simulink model "Latest_HIWI_model"  (R2023b)
settings: Solver=VariableStepAuto  StartTime=0*24*3600  StopTime=24*3600*3  MaxStep=60  RelTol=1e-4  EnableMultiTasking=on
values from neighbouring files (symbols this model uses):
  C_Battery_kWh = 80    [workspaceHIWI.mat]
  discharge_car = [0 3600 7200 10800 14400 18000 21600 25200 28800 32400 36000 39600 ... (146 elements, 73x2)]    [workspaceHIWI.mat]
  Max_charge_potential = 5000    [workspaceHIWI.mat]
  P_Inv_W_max = 12000    [workspaceHIWI.mat]
  PV_W = 10000    [workspaceHIWI.mat]
  ReqSOCandtime1 = [0 3600 7200 10800 14400 18000 21600 25200 28800 32400 36000 39600 ... (219 elements, 73x3)]    [workspaceHIWI.mat]
  SOC_max = 1    [workspaceHIWI.mat]
  SOC_min = 0.1    [workspaceHIWI.mat]
undefined symbols (not defined in the file or in its folder): Davies, Hay, path_carnot, phase
libraries: carnot x11
settings Model: Creator=drhf  LastModifiedBy=Rohan
settings SolverCC: AlgebraicLoopSolver=TrustRegion  EnableFixedStepZeroCrossing=on
settings DataIOCC: LimitDataPoints=on  SaveFormat=Array  ReturnWorkspaceOutputs=off
settings OptimizationCC: ExpressionDepthLimit=2147483647  LifeSpan=inf
settings DebuggingCC: AlgebraicLoopMsg=none  UnderspecifiedInitializationDetection=Classic  MergeDetectMultiDrivingBlocksExec=none  SolverPrmCheckMsg=warning  FcnCallInpInsideContextMsg=warning  UnconnectedInputMsg=warning  UnconnectedOutputMsg=warning  UnconnectedLineMsg=warning  StateNameClashWarn=warning  SFUnexpectedBacktrackingDiag=warning  SFNoUnconditionalDefaultTransitionDiag=warning  SFExecutionAtInitializationDiag=none  ArithmeticOperatorsInVariantConditions=warning
settings HardwareCC: ProdBitPerPointer=32  ProdBitPerSizeT=32  ProdBitPerPtrDiffT=32  ProdLargestAtomicFloat=None  ProdIntDivRoundTo=Undefined  ProdEndianess=Unspecified  ProdWordSize=32  ProdHWDeviceType=32-bit Generic
settings ModelReferenceCC: EnableRefExpFcnMdlSchedulingChecks=on  PropagateSignalLabelsOutOfModel=off
settings SFSimCC: SimUseLocalCustomCode=off  CustomCodeUndefinedFunction=UseInterfaceOnly
settings RTWCC: RTWUseLocalCustomCode=off
settings CodeAppCC: StateflowObjectComments=on
settings GRTTargetCC: TargetLangStandard=C89/C90 (ANSI)  CombineOutputUpdateFcns=off  GRTInterface=on
settings ConfigComp: CovMetricSettings=dw  CovSaveCumulativeToWorkspaceVar=on  CovSaveSingleToWorkspaceVar=on  CovExternalEMLEnable=off

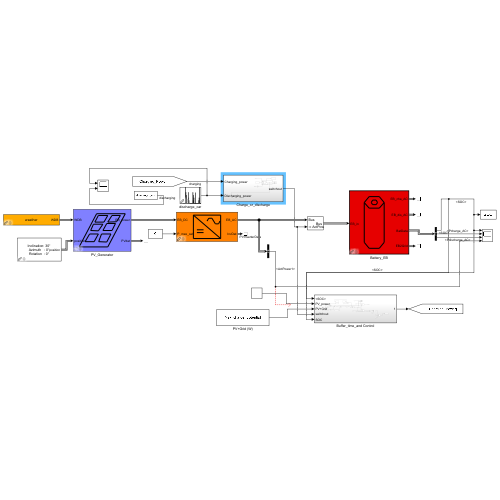
[thumbnail: Simulink's stored preview of the top-level diagram]
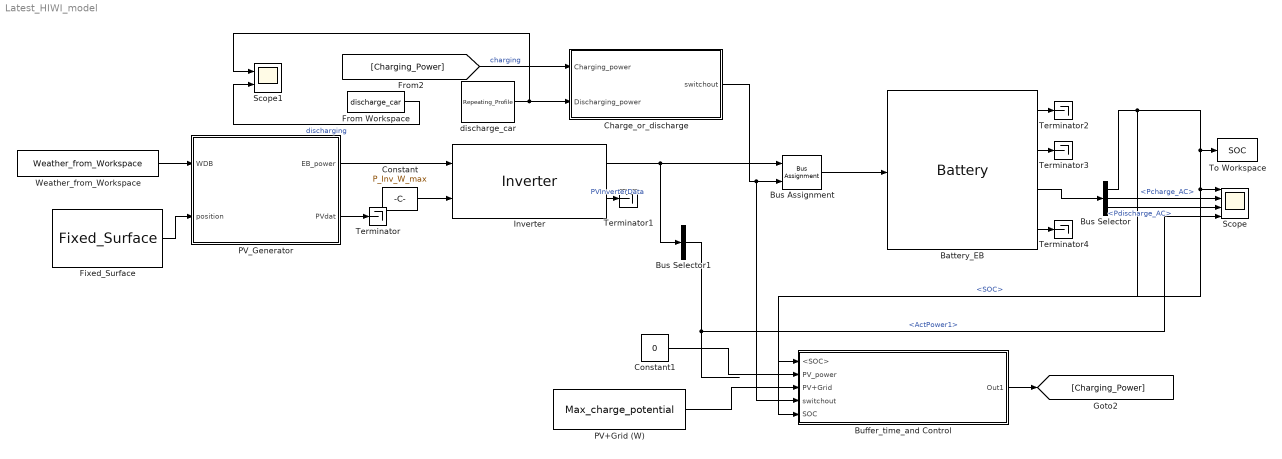
== system Latest_HIWI_model ==
  Battery_EB : carnot/Storage/Electric/Battery  cap_kWh=C_Battery_kWh  eta_ch=n_Charge  eta_dis=n_Discharge  cap0=(SOC_max+SOC_min)/2  SOC_max=SOC_max  SOC_min=SOC_min  Pmax=P_Charge_W  Pmin=P_Discharge_W  P_standby=0
  Buffer_time_and Control : Subsystem
  Bus Assignment : BusAssignment  AssignedSignals=ActPower1
  Bus Selector : BusSelector  OutputSignals=SOC,Pcharge_AC,Pdischarge_AC
  Bus Selector1 : BusSelector  OutputSignals=ActPower1
  Charge_or_discharge : Subsystem
  Constant : Constant  Value=P_Inv_W_max
  Constant1 : Constant  Value=0
  Fixed_Surface : carnot/Weather/Fixed_Surface  colangle=30  colazi=0  colrot=0
  From Workspace : FromWorkspace  VariableName=discharge_car
  Inverter : carnot/Source/Electric_Generator/Inverter  PathName=fullfile(path_carnot('libsl'), 'Source','Electric_Generator','Inverter','parameter_set')  FileName='<user defined>'  userPath=off  userParam=on  Pacnom=P_Inv_W  nphase=1-phase  U=230  f=50  PstepsEta=[0 0.1 0.2 0.25 0.3 0.5 0.75 1]  Eta=[0 0.948 0.966 0.969 0.97 0.972 0.97 0.967]  P_standby=2
  PV+Grid (W) : Constant  Value=Max_charge_potential
  PV_Generator : Subsystem  AncestorBlock=carnot/Source/Electric_Generator/PV_Generator  mask(PV_Module_simple){Wp=PV_W, delta_Wp_K=0.0047, fgen=0.91 % 0.06 power missmatch, 0.01 diodes, 0.02 data sheet tolerance}
      mask prompts: Wp "Peak power of the generator [W]"; delta_Wp_K "Temperature coefficient Pmax 1/K"; fgen "efficiency generator field (lossses in diodes, power missmatch, dirt)"
      mask help:
      | This block simultes a PV module or generatater and calculates the DC power based on the parameters:
      | - Wp of one module or generator at STC [W]
      | - temperature coefficient of Pmax [1/K]
      | - dirt and degradation effects
      | The output DC power of the PV generator is ActPower1 in EB (power only)
      mask Help: web(fullfile(path_carnot('help'),'PV_Generator.html'),'-helpbrowser')
      mask Display: plot(0,0,100,100,[10,40,90,60,10],[10,90,90,10,10],[37,53,60,43,37],[70,70,86,86,70],[60,75,82,67,60],[70,71,86,86,70],[35,30,43,51,35],[65,50,49,65,65],[51,67,73,58,51],[50,50,66,66,50],[28,20,36,43,28],[41,23,23,41,41],[49,44,58,65,49],[41,23,22,41,41])
  Scope : Scope  NumInputPorts=4
  Scope1 : Scope  NumInputPorts=2
  Terminator{,1..4} (5 alike) : Terminator
  To Workspace : ToWorkspace  VariableName=SOC  SampleTime=-1
  Weather_from_Workspace : carnot/Weather/Weather_from_Workspace  file=weather
  discharge_car : carnot/Load/General/Repeating_Profile  period=discharge_car(end,1)  rep_seq_t=discharge_car(:,1)'  rep_seq_d=[1 ]*3600  rep_seq_y=discharge_car(:,2)'
  wires:
  PV_Generator/1(EB_power) -> Inverter/1
  Fixed_Surface/1 -> PV_Generator/2(position)
  Weather_from_Workspace/1 -> PV_Generator/1(WDB)
  PV_Generator/2(PVdat) -> Terminator/1
  Constant/1 -> Inverter/2
  Inverter/2 -> Terminator1/1  "PVInverterData"
  Bus Assignment/1 -> Battery_EB/1
  Inverter/1 -> Bus Selector1/1, Bus Assignment/1
  Battery_EB/3 -> Bus Selector/1
  Bus Selector/1 -> Buffer_time_and Control/5(SOC), Scope/1, To Workspace/1, Buffer_time_and Control/1(<SOC>)  "<SOC>"
  Bus Selector1/1 -> Scope/4  "<ActPower1>"
  Bus Selector/2 -> Scope/2  "<Pcharge_AC>"
  Bus Selector/3 -> Scope/3  "<Pdischarge_AC>"
  Battery_EB/1 -> Terminator2/1
  Battery_EB/2 -> Terminator3/1
  Battery_EB/4 -> Terminator4/1
  Buffer_time_and Control/1(Out1) -> [Charging_Power]
  Charge_or_discharge/1(switchout) -> Buffer_time_and Control/4(switchout), Bus Assignment/2
  [Charging_Power] -> Charge_or_discharge/1(Charging_power)  "charging"
  From Workspace/1 -> Scope1/2  "discharging"
  PV+Grid (W)/1 -> Buffer_time_and Control/3(PV+Grid)
  discharge_car/1 -> Scope1/1, Charge_or_discharge/2(Discharging_power)
  Constant1/1 -> Buffer_time_and Control/2(PV_power)

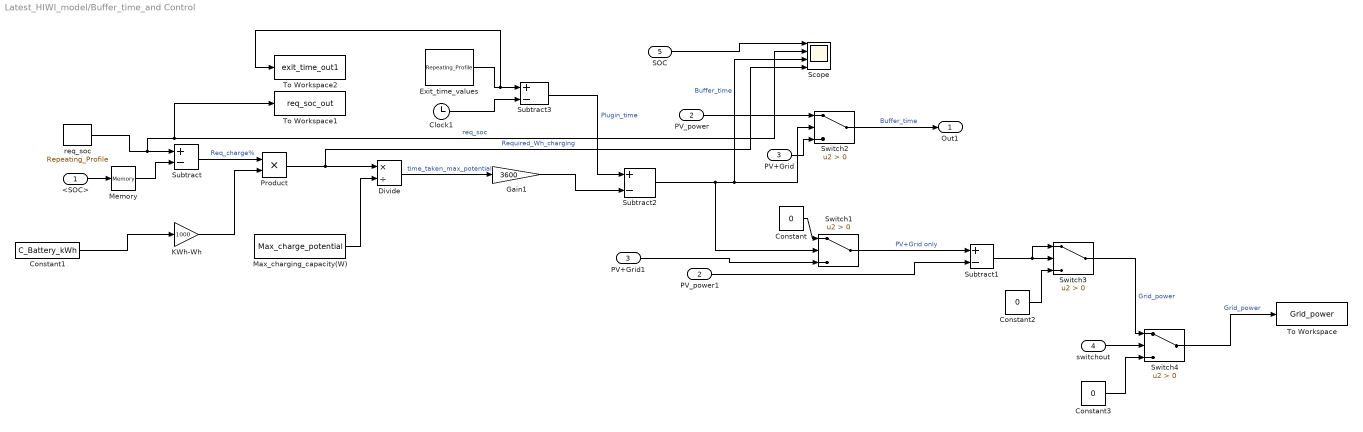
== system Latest_HIWI_model/Buffer_time_and Control ==
  <SOC> : Inport
  PV_power : Inport  Port=2
  PV+Grid : Inport  Port=3
  switchout : Inport  Port=4
  SOC : Inport  Port=5
  Clock1 : Clock
  Constant : Constant  Value=0
  Constant1 : Constant  Value=C_Battery_kWh
  Constant2 : Constant  Value=0
  Constant3 : Constant  Value=0
  Divide : Product  Inputs=*/
  Exit_time_values : carnot/Load/General/Repeating_Profile  period=ReqSOCandtime1(end,1)  rep_seq_t=ReqSOCandtime1(:,1)'  rep_seq_d=[1 ]*3600  rep_seq_y=ReqSOCandtime1(:,3)'
  Gain1 : Gain  Gain=3600
  KWh-Wh : Gain  Gain=1000
  Max_charging_capacity(W) : Constant  Value=Max_charge_potential
  Memory : Memory  InitialCondition=0.55
  PV+Grid1 : InportShadow  Port=3
  PV_power1 : InportShadow  Port=2
  Product : Product
  Scope : Scope  NumInputPorts=4
  Subtract{,1..3} (4 alike) : Sum  Inputs=+-
  Switch{1..4} (4 alike) : Switch  Criteria=u2 > Threshold  SaturateOnIntegerOverflow=off  InputSameDT=off
  To Workspace : ToWorkspace  VariableName=Grid_power  SampleTime=-1
  To Workspace1 : ToWorkspace  VariableName=req_soc_out  SaveFormat=Timeseries  SampleTime=-1
  To Workspace2 : ToWorkspace  VariableName=exit_time_out1  SaveFormat=Timeseries  SampleTime=-1
  req_soc : carnot/Load/General/Repeating_Profile  period=ReqSOCandtime1(end,1)  rep_seq_t=ReqSOCandtime1(:,1)'  rep_seq_d=[1 ]*3600  rep_seq_y=ReqSOCandtime1(:,2)'
  Out1 : Outport
  wires:
  Subtract3/1 -> Subtract2/1  "Plugin_time"
  KWh-Wh/1 -> Product/2
  Max_charging_capacity(W)/1 -> Divide/2
  Subtract2/1 -> Switch1/2, Scope/3, Switch2/2  "Buffer_time"
  Product/1 -> Scope/4, Divide/1  "Required_Wh_charging"
  Subtract/1 -> Product/1  "Req_charge%"
  req_soc/1 -> To Workspace1/1, Scope/2, Subtract/1  "req_soc"
  Exit_time_values/1 -> To Workspace2/1, Subtract3/1
  Gain1/1 -> Subtract2/2
  Divide/1 -> Gain1/1  "time_taken_max_potential"
  Clock1/1 -> Subtract3/2
  Constant1/1 -> KWh-Wh/1
  Switch2/1 -> Out1/1  "Buffer_time"
  <SOC>/1 -> Memory/1
  PV_power/1 -> Switch2/1
  PV+Grid/1 -> Switch2/3
  PV_power1/1 -> Subtract1/2
  PV+Grid1/1 -> Switch1/3
  Subtract1/1 -> Switch3/1, Switch3/2
  Constant2/1 -> Switch3/3
  Switch3/1 -> Switch4/1  "Grid_power"
  Switch1/1 -> Subtract1/1  "PV+Grid only"
  Constant/1 -> Switch1/1
  switchout/1 -> Switch4/2
  Constant3/1 -> Switch4/3
  Switch4/1 -> To Workspace/1  "Grid_power"
  SOC/1 -> Scope/1
  Memory/1 -> Subtract/2

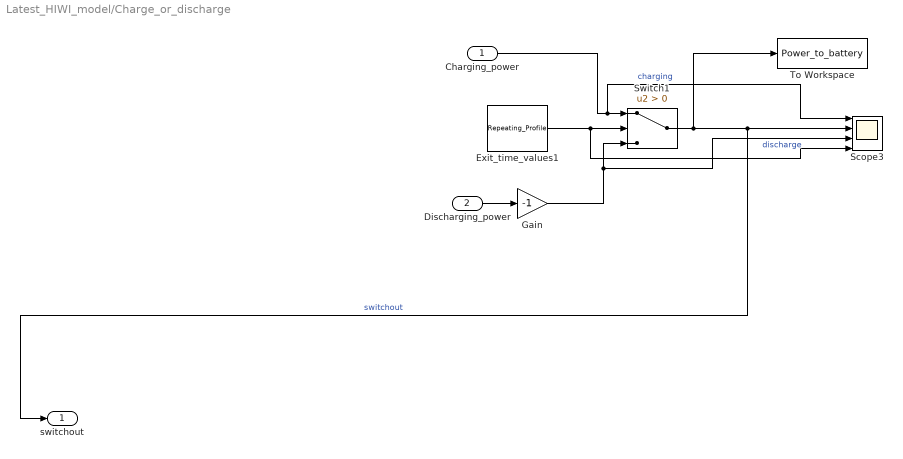
== system Latest_HIWI_model/Charge_or_discharge ==
  Charging_power : Inport
  Discharging_power : Inport  Port=2
  Exit_time_values1 : carnot/Load/General/Repeating_Profile  period=ReqSOCandtime1(end,1)  rep_seq_t=ReqSOCandtime1(:,1)'  rep_seq_d=[1 ]*3600  rep_seq_y=ReqSOCandtime1(:,3)'
  Gain : Gain  Gain=-1
  Scope3 : Scope  NumInputPorts=4
  Switch1 : Switch  Criteria=u2 > Threshold  SaturateOnIntegerOverflow=off  InputSameDT=off  OutDataTypeStr=Inherit: Same as first input
  To Workspace : ToWorkspace  VariableName=Power_to_battery  SaveFormat=Timeseries  SampleTime=-1
  switchout : Outport
  wires:
  Switch1/1 -> To Workspace/1, switchout/1, Scope3/2  "switchout"
  Charging_power/1 -> Scope3/1, Switch1/1  "charging"
  Exit_time_values1/1 -> Scope3/4, Switch1/2
  Gain/1 -> Scope3/3, Switch1/3  "discharge"
  Discharging_power/1 -> Gain/1

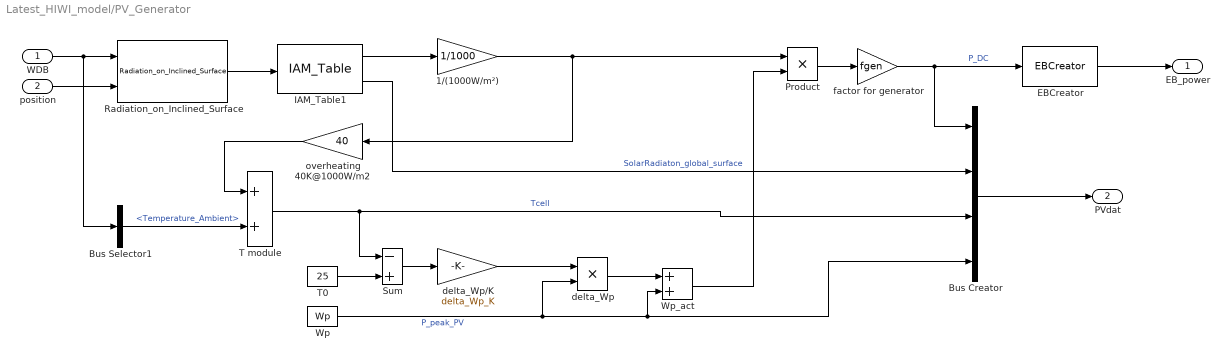
== system Latest_HIWI_model/PV_Generator ==
  WDB : Inport
  position : Inport  Port=2
  1/(1000W/m²) : Gain  Gain=1/1000
  Bus Creator : BusCreator  Inputs=4
  Bus Selector1 : BusSelector  OutputSignals=Temperature_Ambient
  EBCreator : carnot/Basic/Electric/EBCreator  Inport_ID=off  Inport_f=off  Inport_v1=off  Inport_p1=on  Inport_pf1=off  Inport_v2=off  Inport_p2=off  Inport_pf2=off  Inport_v3=off  Inport_p3=off  Inport_pf3=off  ID=1  f=0  v1=0  p1=1e5  pf1=1  v2=0  p2=0  pf2=0  v3=0  p3=0  pf3=0  Annotation_ID=off  Annotation_f=off  Annotation_v1=off  Annotation_p1=off  Annotation_pf1=off  Annotation_v2=off  Annotation_p2=off  Annotation_pf2=off  Annotation_v3=off  Annotation_p3=off  Annotation_pf3=off
  IAM_Table1 : carnot/Source/Solar_Thermal/IncidenceAngleModifier/IAM_Table  fta=1  angle=[0:5:90]  Kb="[1.0000    1.0000    0.9999    0.9996    0.9991    0.9982    0.9965  0.9935    0.9886    0.9807    0.9678    0.9473    0.9148    0.8638   0.7846    0.6644    0.4907    0.2599    0.0000]"  Kd=0.915
  Product : Product  RndMeth=Zero
  Radiation_on_Inclined_Surface : carnot/Weather/Radiation_on_Inclined_Surface  sky=Hay-Davies  reflect=0.2
  Sum : Sum  Inputs=-+
  T module : Sum  Inputs=2
  T0 : Constant  Value=25
  Wp : Constant  Value=Wp
  Wp_act : Sum
  delta_Wp : Product  RndMeth=Zero
  delta_Wp/K : Gain  Gain=delta_Wp_K
  factor for generator : Gain  Gain=fgen
  overheating 40K@1000W/m2 : Gain  Gain=40
  EB_power : Outport  VectorParamsAs1DForOutWhenUnconnected=off
  PVdat : Outport  Port=2  VectorParamsAs1DForOutWhenUnconnected=off
  wires:
  IAM_Table1/2 -> Bus Creator/2  "SolarRadiaton_global_surface"
  position/1 -> Radiation_on_Inclined_Surface/2
  Radiation_on_Inclined_Surface/1 -> IAM_Table1/1
  WDB/1 -> Radiation_on_Inclined_Surface/1, Bus Selector1/1
  factor for generator/1 -> EBCreator/1, Bus Creator/1  "P_DC"
  delta_Wp/K/1 -> delta_Wp/1
  Product/1 -> factor for generator/1
  1/(1000W/m²)/1 -> Product/1, overheating 40K@1000W/m2/1
  Wp_act/1 -> Product/2
  T module/1 -> Sum/1, Bus Creator/3  "Tcell"
  IAM_Table1/1 -> 1/(1000W/m²)/1
  T0/1 -> Sum/2
  Sum/1 -> delta_Wp/K/1
  overheating 40K@1000W/m2/1 -> T module/1
  Bus Selector1/1 -> T module/2  "<Temperature_Ambient>"
  Wp/1 -> Wp_act/2, Bus Creator/4, delta_Wp/2  "P_peak_PV"
  delta_Wp/1 -> Wp_act/1
  Bus Creator/1 -> PVdat/1
  EBCreator/1 -> EB_power/1
